simulink model "Bitwise_Operater"  (R2023b)
settings: Solver=VariableStepAuto  StartTime=0.0  StopTime=10.0  RelTol=1e-3
libraries: simulink x3
settings Model: Creator=hp  LastModifiedBy=hp

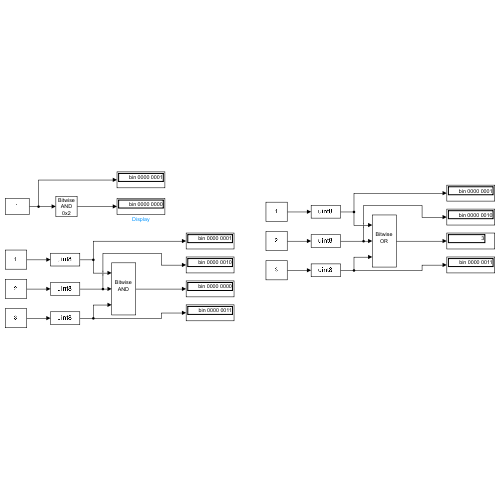
[thumbnail: Simulink's stored preview of the top-level diagram]
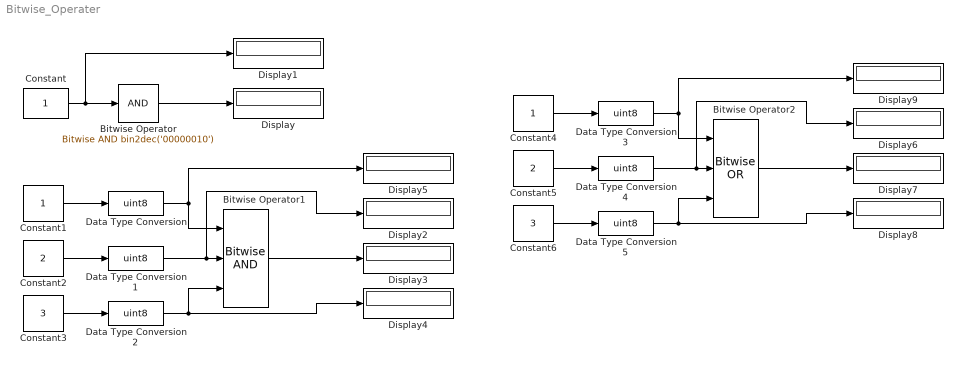
== system Bitwise_Operater ==
  Bitwise Operator : simulink/Logic and Bit Operations/Bitwise Operator  logicop=AND  UseBitMask=on  BitMask=bin2dec('00000010')  BitMaskRealWorld=Stored Integer
  Bitwise Operator1 : simulink/Logic and Bit Operations/Bitwise Operator  logicop=AND  UseBitMask=off  NumInputPorts=3  BitMask=bin2dec('00000010')  BitMaskRealWorld=Stored Integer
  Bitwise Operator2 : simulink/Logic and Bit Operations/Bitwise Operator  logicop=OR  UseBitMask=off  NumInputPorts=3  BitMask=bin2dec('00000010')  BitMaskRealWorld=Stored Integer
  Constant : Constant  OutDataTypeStr=uint8
  Constant1 : Constant
  Constant2 : Constant  Value=2
  Constant3 : Constant  Value=3
  Constant4 : Constant
  Constant5 : Constant  Value=2
  Constant6 : Constant  Value=3
  Data Type Conversion{,1..5} (6 alike) : DataTypeConversion  OutDataTypeStr=uint8  SaturateOnIntegerOverflow=off  RndMeth=Floor
  Display{,1..9} (10 alike) : Display
      Display settings: Format=binary (Stored Integer)
      Display1 settings: Format=binary (Stored Integer)
      Display2 settings: Format=binary (Stored Integer)
      Display3 settings: Format=binary (Stored Integer)
      Display4 settings: Format=binary (Stored Integer)
      Display5 settings: Format=binary (Stored Integer)
      Display6 settings: Format=binary (Stored Integer)
      Display8 settings: Format=binary (Stored Integer)
      Display9 settings: Format=binary (Stored Integer)
  wires:
  Constant/1 -> Display1/1, Bitwise Operator/1
  Bitwise Operator/1 -> Display/1
  Bitwise Operator1/1 -> Display3/1
  Constant1/1 -> Data Type Conversion/1
  Constant2/1 -> Data Type Conversion1/1
  Constant3/1 -> Data Type Conversion2/1
  Data Type Conversion/1 -> Display5/1, Bitwise Operator1/1
  Data Type Conversion1/1 -> Display2/1, Bitwise Operator1/2
  Data Type Conversion2/1 -> Display4/1, Bitwise Operator1/3
  Data Type Conversion5/1 -> Bitwise Operator2/3, Display8/1
  Data Type Conversion4/1 -> Bitwise Operator2/2, Display6/1
  Data Type Conversion3/1 -> Bitwise Operator2/1, Display9/1
  Constant6/1 -> Data Type Conversion5/1
  Constant5/1 -> Data Type Conversion4/1
  Constant4/1 -> Data Type Conversion3/1
  Bitwise Operator2/1 -> Display7/1
